simulink model "GPSIMUSignals"  (R2024b)
settings: Solver=FixedStepAuto  StartTime=0.0  StopTime=10.0  RelTol=1e-3
settings Model: DataDictionary=Master_Dictionary.sldd  EnableAccessToBaseWorkspace=off  Creator=torni  LastModifiedBy=will
settings SolverCC: AlgebraicLoopSolver=TrustRegion
settings DataIOCC: ReturnWorkspaceOutputs=off
settings OptimizationCC: DefaultParameterBehavior=Inlined  EnhancedBackFolding=on  PassReuseOutputArgsAs=Individual arguments  ZeroExternalMemoryAtStartup=off  ZeroInternalMemoryAtStartup=off  OptimizeBlockOrder=speed  DifferentSizesBufferReuse=on  OptimizationCustomize=off  EfficientTunableParamExpr=on
settings DebuggingCC: ParameterTunabilityLossMsg=error  UnconnectedInputMsg=warning  UnconnectedOutputMsg=warning  UnconnectedLineMsg=warning  ArithmeticOperatorsInVariantConditions=warning
settings HardwareCC: TargetLargestAtomicInteger=Long  TargetLargestAtomicFloat=Double  TargetIntDivRoundTo=Zero  TargetEndianess=LittleEndian  TargetHWDeviceType=ARM Compatible->ARM Cortex-M  ProdEqTarget=off
settings ModelReferenceCC: EnableRefExpFcnMdlSchedulingChecks=on
settings SFSimCC: MATLABDynamicMemAlloc=off  CustomCodeUndefinedFunction=UseInterfaceOnly
settings RTWCC: Description=Embedded Coder  SystemTargetFile=ert.tlc  TemplateMakefile=ert_default_tmf  Toolchain=GNU Tools for ARM Embedded Processors  RTWCompilerOptimization=on  GPUComputeCapability=3.5
settings CodeAppCC: ForceParamTrailComments=on  IgnoreCustomStorageClasses=off  OperatorAnnotations=on  SimulinkDataObjDesc=on  SFDataObjDesc=on  InsertBlockDesc=on
settings ERTTargetCC: TargetLangStandard=C99 (ISO)  GenerateSampleERTMain=on  ERTCustomFileTemplate=example_file_process.tlc

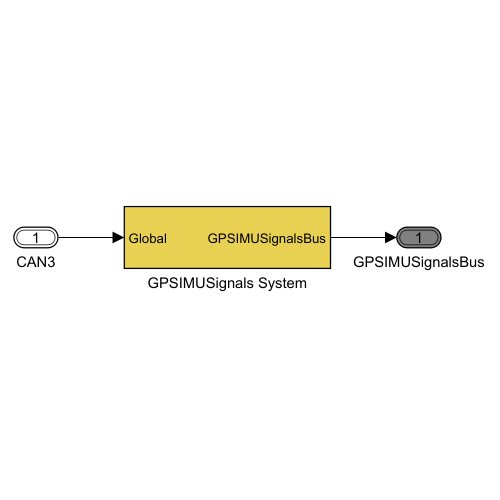
[thumbnail: Simulink's stored preview of the top-level diagram]
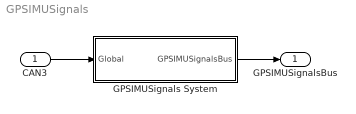
== system GPSIMUSignals ==
  CAN3 : Inport  OutDataTypeStr=Bus: CAN3Bus
  GPSIMUSignals System : Subsystem
  GPSIMUSignalsBus : Outport  OutDataTypeStr=Bus: GPSIMUSignalsBus  VectorParamsAs1DForOutWhenUnconnected=off
  wires:
  CAN3/1 -> GPSIMUSignals System/1(Global)
  GPSIMUSignals System/1(GPSIMUSignalsBus) -> GPSIMUSignalsBus/1

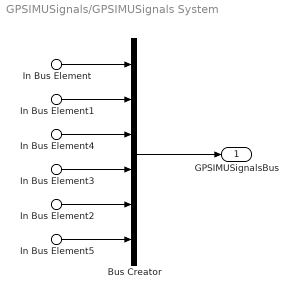
== system GPSIMUSignals/GPSIMUSignals System ==
  In Bus Element : Inport  PortName=Global  Element=GPSIMUSignalsBus.vLateralOXTSIMU
  In Bus Element1 : Inport  PortName=Global  Element=GPSIMUSignalsBus.gVerticalOXTSIMU
  In Bus Element3 : Inport  PortName=Global  Element=GPSIMUSignalsBus.gLateralOXTSIMU
  In Bus Element4 : Inport  PortName=Global  Element=GPSIMUSignalsBus.vLongitudinalOXTS
  In Bus Element2 : Inport  PortName=Global  Element=GPSIMUSignalsBus.gLongitudinalOXTS
  In Bus Element5 : Inport  PortName=Global  Element=GPSIMUSignalsBus.dnYawAccelOXTS
  Bus Creator : BusCreator  Inputs=6  OutDataTypeStr=Bus: GPSIMUSignalsBus
  GPSIMUSignalsBus : Outport  OutDataTypeStr=Bus: GPSIMUSignalsBus  VectorParamsAs1DForOutWhenUnconnected=off
  wires:
  Bus Creator/1 -> GPSIMUSignalsBus/1
  In Bus Element/1 -> Bus Creator/1
  In Bus Element1/1 -> Bus Creator/2
  In Bus Element4/1 -> Bus Creator/3
  In Bus Element3/1 -> Bus Creator/4
  In Bus Element2/1 -> Bus Creator/5
  In Bus Element5/1 -> Bus Creator/6
